simulink model "gm_CustArch_v7_vnl"  (R2020a)
settings: Solver=FixedStepDiscrete  StartTime=0.0  StopTime=840000  RelTol=1e-3
libraries: simulink x175, hdlsllib x114, hdlmdlgenlib x2
(part 2 of 4)

== system gm_CustArch_v7_vnl/cust_architecture_vnl/collect_output/read_from_magic_and_timestamp ==
  note: This subsystem in needed for save in a specific RAM the magic number
      | and the timestamp
  OutputState : Inport
  FIFO_data_in : Inport  Port=2
  FIFO_write_to : Inport  Port=3
  InputState : Inport  Port=4
  Terminator1 : Terminator
  getting address and enable for Magic and Timestamps : Subsystem
  input_RAM_for_MagicNumber_TimeStamps : hdlsllib/HDL RAMs/Dual Port RAM  ram_size=8
      settings: SourceProductBaseCode=SL
  read_from_Magic_TS : Outport
  wires:
  FIFO_write_to/1 -> getting address and enable for Magic and Timestamps/2(FIFO_write_to)
  InputState/1 -> getting address and enable for Magic and Timestamps/1(InputState)
  OutputState/1 -> input_RAM_for_MagicNumber_TimeStamps/4
  input_RAM_for_MagicNumber_TimeStamps/1 -> Terminator1/1
  getting address and enable for Magic and Timestamps/1(wr_address) -> input_RAM_for_MagicNumber_TimeStamps/2
  input_RAM_for_MagicNumber_TimeStamps/2 -> read_from_Magic_TS/1  "read_from_Magic_TS"
  getting address and enable for Magic and Timestamps/2(wr_enable) -> input_RAM_for_MagicNumber_TimeStamps/3
  FIFO_data_in/1 -> input_RAM_for_MagicNumber_TimeStamps/1

== system gm_CustArch_v7_vnl/cust_architecture_vnl/input_interpret_store_retrieve/Interpret_to_RAM_input ==
  note: These subsystems identify the sources of the incoming data (amplifier --> source_device and channel number) and
      | determine the address to be associated to the current data for the RAM storage. This statement is valid for all the kind of
      | data except for the magic number and the timestamp that are directly sent to a different RAM in the Output section
  FIFO_data_in : Inport
  FIFO_write_to : Inport  Port=2
  InputState : Inport  Port=3
  data_stream_enable : Inport  Port=4
  RAM address definition : Subsystem
  interpret incoming data : Subsystem
  device_output : Outport
  inc_source_device : Outport  Port=2
  wr_din : Outport  Port=3
  write address : Outport  Port=4
  wr_en : Outport  Port=5
  wires:
  RAM address definition/1(wr_din) -> wr_din/1  "wr_din"
  RAM address definition/2(wr_addr) -> write address/1  "write address"
  FIFO_data_in/1 -> RAM address definition/1(DataIn)
  FIFO_write_to/1 -> interpret incoming data/1(FIFO_write_to), RAM address definition/6(write_to)
  interpret incoming data/5(converter_cnt) -> RAM address definition/5(converter_cnt)
  InputState/1 -> interpret incoming data/2(InputState), RAM address definition/2(InputState)
  interpret incoming data/3(device_output) -> device_output/1
  RAM address definition/3(write_enable_6to15) -> wr_en/1  "wr_en"
  data_stream_enable/1 -> interpret incoming data/3(data_stream_enable)
  interpret incoming data/1(source_device) -> RAM address definition/4(source_device)
  interpret incoming data/2(inc_source_device) -> inc_source_device/1
  interpret incoming data/4(source_channel_0_159) -> RAM address definition/3(source_channel_0_159)

== system gm_CustArch_v7_vnl/cust_architecture_vnl/input_interpret_store_retrieve/store_and_retrieve_input ==
  note: address sent for processing
  note: data sent for processing
  note: reading address
      | from output
  note: current data
  note: current data
  note: Two dual-port RAM for storage and processing
  note: this memory is for synchronizing the current value and
      | the read_from_porcessing_addr since to ouput a value
      | the dual port RAM needs a single clock
  note: writing address
  note: data sent to Output
  read address : Inport
  wr_din : Inport  Port=2
  wr_address : Inport  Port=3
  wr_en : Inport  Port=4
  Memory4 : Memory  InheritSampleTime=on
  Terminator : Terminator
  Terminator6 : Terminator
  input_storage : hdlsllib/HDL RAMs/Dual Port RAM  ram_size=9
      settings: SourceProductBaseCode=SL
  input_storage_for_processing : hdlsllib/HDL RAMs/Dual Port RAM  ram_size=9
      settings: SourceProductBaseCode=SL
  read_from_storage_value : Outport
  current_value : Outport  Port=2
  read_from_porcessing_addr : Outport  Port=3
  wires:
  input_storage_for_processing/2 -> current_value/1  "current value"
  input_storage/2 -> read_from_storage_value/1  "read_from_storage"
  wr_din/1 -> input_storage/1, input_storage_for_processing/1
  input_storage_for_processing/1 -> Terminator6/1
  wr_en/1 -> input_storage/3, input_storage_for_processing/3
  input_storage/1 -> Terminator/1
  read address/1 -> input_storage/4
  wr_address/1 -> input_storage/2, input_storage_for_processing/2, Memory4/1
  Memory4/1 -> input_storage_for_processing/4, read_from_porcessing_addr/1  "read from porcessing addr"

== system gm_CustArch_v7_vnl/cust_architecture_vnl/output_interpret/Interpret_to_RAM_output ==
  OutputState : Inport
  data_stream_en : Inport  Port=2
  Output_State_to_RAM_address (to read) : Subsystem
  "get_enabled_timings " : Subsystem  MinMaxOverflowLogging=MinMaxAndOverflow
  rd_enable : Outport
  read address : Outport  Port=2
  wires:
  Output_State_to_RAM_address (to read)/1(rd_enable) -> rd_enable/1
  data_stream_en/1 -> "get_enabled_timings "/2(data_stream_en)
  OutputState/1 -> "get_enabled_timings "/1(OutputState), Output_State_to_RAM_address (to read)/3(OutputState)
  "get_enabled_timings "/1(source_channel_en) -> Output_State_to_RAM_address (to read)/1(source_channel_en)
  "get_enabled_timings "/2(source_channel_0_159) -> Output_State_to_RAM_address (to read)/2(source_channel_0_159)
  "get_enabled_timings "/3(source_device_enabled) -> Output_State_to_RAM_address (to read)/4(source_device_en)
  Output_State_to_RAM_address (to read)/2(rd_addr) -> read address/1
  "get_enabled_timings "/4(source_device) -> Output_State_to_RAM_address (to read)/5(source_device)
  "get_enabled_timings "/5(converter_cnt) -> Output_State_to_RAM_address (to read)/6(converter_cnt)

== system gm_CustArch_v7_vnl/cust_architecture_vnl/process_and_retrieve/digital_filter ==
  current_sample : Inport  OutDataTypeStr=fixdt(0,16,0)
  previous_sample : Inport  Port=2
  Enable : EnablePort
  Constant : Constant  Value=32768  OutDataTypeStr=fixdt(0,16,0)  SampleTime=-1
  Constant1 : Constant  Value=32768  OutDataTypeStr=fixdt(0,16,0)  SampleTime=-1
  HP_Butter_2nd : Subsystem  Tag=FilterWizardSubSystem
      settings: ErrorFcn=dspFilterRealizedInBasicElemsAlgLoopErrFcnCallback
  Subtract : Sum  Inputs=+-  OutDataTypeStr=fixdt(1,16,4)
  Subtract1 : Sum  OutDataTypeStr=fixdt(0,16,0)
  filter_output : Outport  InitialOutput=[0]
  new_previous_sample : Outport  Port=2  InitialOutput=[0]
  wires:
  HP_Butter_2nd/2(Output1) -> new_previous_sample/1
  previous_sample/1 -> HP_Butter_2nd/2(Input1)
  Subtract1/1 -> filter_output/1
  Constant1/1 -> Subtract1/2
  HP_Butter_2nd/1(Output) -> Subtract1/1
  current_sample/1 -> Subtract/1
  Subtract/1 -> HP_Butter_2nd/1(Input)
  Constant/1 -> Subtract/2

== system gm_CustArch_v7_vnl/cust_architecture_vnl/process_and_retrieve/previous_sample_storage1 ==
  note: ritardo scrittura su data2 1 campione
  new_previous_sample : Inport
  input_state_AC_TRUE-3 : Inport  Port=2
  write porcessing addr = read from storage addr +1 : Inport  Port=3
  input_state_AC_TRUE : Inport  Port=4
  1st : Constant  OutDataTypeStr=boolean  SampleTime=-1
  Bit Concat : hdlsllib/Logic and Bit Operations/Bit Concat  numInputs=2
  Compare To Constant2 : simulink/Logic and Bit Operations/Compare To Constant  relop===  const=1  OutDataTypeStr=boolean
  Delay1 : Delay  DelayLength=1  InitialCondition=0
  Delay4 : Delay  DelayLength=1  InitialCondition=0
  Mux : Mux  Inputs=2
  PreviousData1_storage : hdlsllib/HDL RAMs/Dual Port RAM  ram_size=10
      settings: SourceProductBaseCode=SL
  PreviousData1_storage1 : hdlsllib/HDL RAMs/Dual Port RAM  ram_size=10
      settings: SourceProductBaseCode=SL
  PreviousData_read : Subsystem
  ReadingStateMachine : Stateflow chart  TreatAsAtomicUnit=on
  Terminator1 : Terminator
  Terminator2 : Terminator
  previous_sample : Outport
  wires:
  Delay1/1 -> PreviousData1_storage1/2
  Delay4/1 -> PreviousData1_storage1/3
  PreviousData1_storage1/1 -> Terminator2/1
  Mux/1 -> previous_sample/1
  PreviousData1_storage1/2 -> Mux/1
  Compare To Constant2/1 -> Delay4/1, PreviousData_read/Enable
  ReadingStateMachine/1(StarReading) -> Compare To Constant2/1
  input_state_AC_TRUE/1 -> ReadingStateMachine/1(read_enable)
  PreviousData_read/1(y) -> PreviousData1_storage/4, PreviousData1_storage1/4
  write porcessing addr = read from storage addr +1/1 -> PreviousData_read/1(u2), Bit Concat/2
  input_state_AC_TRUE-3/1 -> PreviousData1_storage/3
  1st/1 -> Bit Concat/1
  PreviousData1_storage/2 -> Mux/2, PreviousData1_storage1/1
  new_previous_sample/1 -> PreviousData1_storage/1
  PreviousData1_storage/1 -> Terminator1/1
  Bit Concat/1 -> PreviousData1_storage/2, Delay1/1

== system gm_CustArch_v7_vnl/cust_architecture_vnl/process_and_retrieve/previous_sample_storage2 ==
  note: ritardo scrittura su data2 1 campione
  new_previous_sample : Inport
  input_state_AC_TRUE : Inport  Port=2
  write porcessing addr = read from storage addr +1 : Inport  Port=3
  1st : Constant  OutDataTypeStr=boolean  SampleTime=-1
  Bit Concat : hdlsllib/Logic and Bit Operations/Bit Concat  numInputs=2
  Constant : Constant  Value=0  OutDataTypeStr=boolean  SampleTime=-1
  Delay : Delay  DelayLength=3  InitialCondition=0
  Delay{1..2,4..5} (4 alike) : Delay  DelayLength=1  InitialCondition=0
  Delay3 : Delay  DelayLength=3  InitialCondition=0
  Detect Change : simulink/Logic and Bit Operations/Detect Change  vinit=0  OutDataTypeStr=boolean
  Mux : Mux  Inputs=2
  PreviousData1_storage : hdlsllib/HDL RAMs/Dual Port RAM  ram_size=10
      settings: SourceProductBaseCode=SL
  PreviousData1_storage1 : hdlsllib/HDL RAMs/Dual Port RAM  ram_size=10
      settings: SourceProductBaseCode=SL
  PreviousData_read : Subsystem
  ReadingStateMachine : Stateflow chart  Commented=on  TreatAsAtomicUnit=on
  Switch : Switch  Criteria=u2 > Threshold
  Terminator1 : Terminator
  Terminator2 : Terminator
  previous_sample : Outport
  wires:
  Switch/1 -> PreviousData1_storage/4, PreviousData1_storage1/4, Delay4/1
  PreviousData_read/1(y) -> Detect Change/1, Switch/1
  Detect Change/1 -> Switch/2
  Constant/1 -> Switch/3
  Mux/1 -> previous_sample/1
  PreviousData1_storage1/2 -> Mux/1
  Delay5/1 -> PreviousData1_storage1/3
  PreviousData1_storage/2 -> PreviousData1_storage1/1, Mux/2
  PreviousData1_storage1/1 -> Terminator2/1
  Delay4/1 -> PreviousData1_storage1/2
  Delay3/1 -> Bit Concat/2
  Delay2/1 -> PreviousData_read/1(u2)
  Delay1/1 -> PreviousData_read/Enable, Delay5/1
  Delay/1 -> PreviousData1_storage/3
  write porcessing addr = read from storage addr +1/1 -> Delay3/1, Delay2/1
  input_state_AC_TRUE/1 -> Delay/1, Delay1/1
  1st/1 -> Bit Concat/1
  new_previous_sample/1 -> PreviousData1_storage/1
  PreviousData1_storage/1 -> Terminator1/1
  Bit Concat/1 -> PreviousData1_storage/2

== system gm_CustArch_v7_vnl/cust_architecture/collect_output/read_from_magic_and_timestamp/getting address and enable for Magic and Timestamps ==
  note: enable the RAM writing if the InputState is between 0 and 5
  InputState : Inport  OutDataTypeStr=uint8  PortDimensions=1  SampleTime=1
  FIFO_write_to : Inport  Port=2  OutDataTypeStr=boolean  PortDimensions=1  SampleTime=1
  AND1 : Logic  AllPortsSameDT=off  OutDataTypeStr=boolean  SampleTime=1
  Compare To Constant10 : simulink/Logic and Bit Operations/Compare To Constant  relop===  const="fi(0,0,8,0,\"hex\",\"04\")"  OutDataTypeStr=boolean
  Compare To Constant11 : simulink/Logic and Bit Operations/Compare To Constant  relop===  const="fi(0,0,8,0,\"hex\",\"05\")"  OutDataTypeStr=boolean
  Compare To Constant12 : simulink/Logic and Bit Operations/Compare To Constant  relop=<=  const="fi(0,0,8,0,\"hex\",\"05\")"  OutDataTypeStr=boolean
  Compare To Constant6 : simulink/Logic and Bit Operations/Compare To Constant  relop===  const="fi(0,0,8,0,\"hex\",\"00\")"  OutDataTypeStr=boolean
  Compare To Constant7 : simulink/Logic and Bit Operations/Compare To Constant  relop===  const="fi(0,0,8,0,\"hex\",\"01\")"  OutDataTypeStr=boolean
  Compare To Constant8 : simulink/Logic and Bit Operations/Compare To Constant  relop===  const="fi(0,0,8,0,\"hex\",\"02\")"  OutDataTypeStr=boolean
  Compare To Constant9 : simulink/Logic and Bit Operations/Compare To Constant  relop===  const="fi(0,0,8,0,\"hex\",\"03\")"  OutDataTypeStr=boolean
  Constant10 : Constant  Value=3  OutDataTypeStr=uint8  SampleTime=1
  Constant11 : Constant  Value=4  OutDataTypeStr=uint8  SampleTime=1
  Constant12 : Constant  Value=5  OutDataTypeStr=uint8  SampleTime=1
  Constant13 : Constant  Value=6  OutDataTypeStr=uint8  SampleTime=1
  Constant7 : Constant  Value=0  OutDataTypeStr=uint8  SampleTime=1
  Constant8 : Constant  OutDataTypeStr=uint8  SampleTime=1
  Constant9 : Constant  Value=2  OutDataTypeStr=uint8  SampleTime=1
  Switch{6..11} (6 alike) : Switch  Criteria=u2 > Threshold  Threshold=double(0)  OutDataTypeStr=uint8  SampleTime=1
  wr_address : Outport  VectorParamsAs1DForOutWhenUnconnected=off
  wr_enable : Outport  Port=2  VectorParamsAs1DForOutWhenUnconnected=off
  wires:
  Switch9/1 -> Switch8/3
  Switch8/1 -> Switch7/3
  Switch7/1 -> Switch6/3
  Switch6/1 -> wr_address/1
  Switch11/1 -> Switch10/3
  Switch10/1 -> Switch9/3
  Constant9/1 -> Switch8/1
  Constant8/1 -> Switch7/1
  Constant7/1 -> Switch6/1
  Constant13/1 -> Switch11/3
  Constant12/1 -> Switch11/1
  Constant11/1 -> Switch10/1
  Constant10/1 -> Switch9/1
  Compare To Constant9/1 -> Switch9/2
  Compare To Constant8/1 -> Switch8/2
  Compare To Constant7/1 -> Switch7/2
  Compare To Constant6/1 -> Switch6/2
  Compare To Constant12/1 -> AND1/1
  Compare To Constant11/1 -> Switch11/2
  Compare To Constant10/1 -> Switch10/2
  AND1/1 -> wr_enable/1
  FIFO_write_to/1 -> AND1/2
  InputState/1 -> Compare To Constant10/1, Compare To Constant11/1, Compare To Constant12/1, Compare To Constant6/1, Compare To Constant7/1, Compare To Constant8/1, Compare To Constant9/1

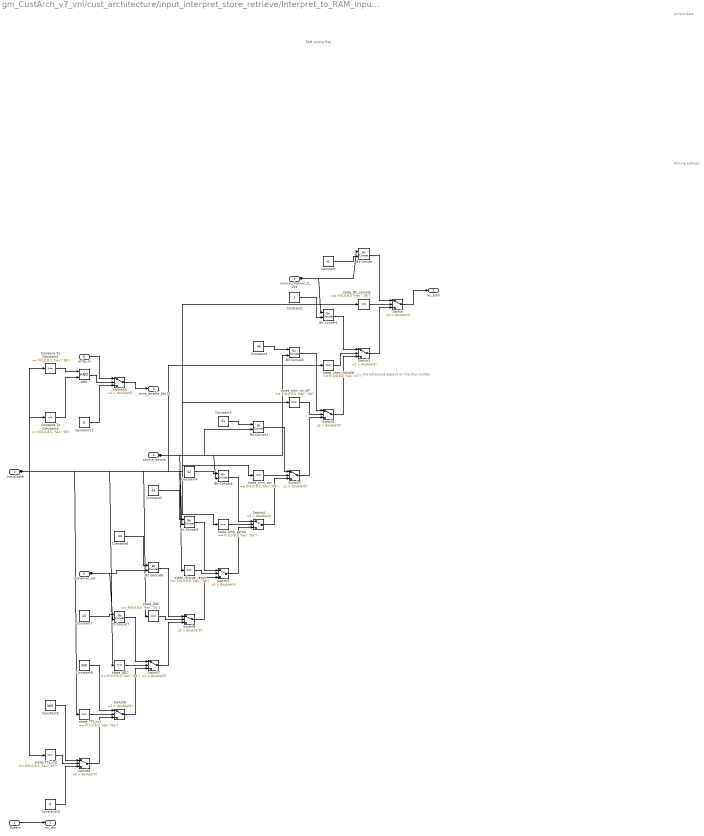
== system gm_CustArch_v7_vnl/cust_architecture/input_interpret_store_retrieve/Interpret_to_RAM_input/RAM address definition ==
  note: RAM writing flag
  note: current data
  note: Writing address
  note: the adressess depend on the chip number
  DataIn : Inport  OutDataTypeStr=uint16  PortDimensions=1  SampleTime=1
  InputState : Inport  Port=2  OutDataTypeStr=uint8  PortDimensions=1  SampleTime=1
  source_channel_0_159 : Inport  Port=3  OutDataTypeStr=uint8  PortDimensions=1  SampleTime=1
  source_device : Inport  Port=4  OutDataTypeStr=fixdt(0, 3, 0)  PortDimensions=1  SampleTime=1
  converter_cnt : Inport  Port=5  OutDataTypeStr=fixdt(0, 3, 0)  PortDimensions=1  SampleTime=1
  write_to : Inport  Port=6  OutDataTypeStr=boolean  PortDimensions=1  SampleTime=1
  AND : Logic  AllPortsSameDT=off  OutDataTypeStr=boolean  SampleTime=1
  Bit Concat{,1..7} (8 alike) : hdlsllib/Logic and Bit Operations/Bit Concat  numInputs=2
  Compare To Constant2 : simulink/Logic and Bit Operations/Compare To Constant  relop=>=  const="fi(0,0,8,0,\"hex\",\"06\")"  OutDataTypeStr=boolean
  Compare To Constant3 : simulink/Logic and Bit Operations/Compare To Constant  relop=<=  const="fi(0,0,8,0,\"hex\",\"0f\")"  OutDataTypeStr=boolean
  Constant : Constant  Value=0  OutDataTypeStr=boolean  SampleTime=1
  Constant1 : Constant  OutDataTypeStr=boolean  SampleTime=1
  Constant10 : Constant  Value=0  OutDataTypeStr=fixdt(0, 9, 1000)  SampleTime=1
  Constant11 : Constant  Value=0  OutDataTypeStr=boolean  SampleTime=1
  Constant2 : Constant  Value=40  OutDataTypeStr=fixdt(0, 6, 0)  SampleTime=1
  Constant3 : Constant  Value=41  OutDataTypeStr=fixdt(0, 6, 0)  SampleTime=1
  Constant4 : Constant  Value=42  OutDataTypeStr=fixdt(0, 6, 0)  SampleTime=1
  Constant5 : Constant  Value=43  OutDataTypeStr=fixdt(0, 6, 0)  SampleTime=1
  Constant6 : Constant  Value=44  OutDataTypeStr=fixdt(0, 6, 0)  SampleTime=1
  Constant7 : Constant  Value=45  OutDataTypeStr=fixdt(0, 6, 0)  SampleTime=1
  Constant8 : Constant  Value=368  OutDataTypeStr=fixdt(0, 9, 0)  SampleTime=1
  Constant9 : Constant  Value=369  OutDataTypeStr=fixdt(0, 9, 0)  SampleTime=1
  Switch{,1..9} (10 alike) : Switch  Criteria=u2 > Threshold  Threshold=double(0)  OutDataTypeStr=fixdt(0, 9, 0)  SampleTime=1
  Switch10 : Switch  Criteria=u2 > Threshold  Threshold=double(0)  OutDataTypeStr=boolean  SampleTime=1
  state_ADC : simulink/Logic and Bit Operations/Compare To Constant  relop===  const="fi(0,0,8,0,\"hex\",\"0d\")"  OutDataTypeStr=boolean
  state_DAC : simulink/Logic and Bit Operations/Compare To Constant  relop===  const="fi(0,0,8,0,\"hex\",\"0c\")"  OutDataTypeStr=boolean
  state_DC_sample : simulink/Logic and Bit Operations/Compare To Constant  relop===  const="fi(0,0,8,0,\"hex\",\"06\")"  OutDataTypeStr=boolean
  state_TTL_in1 : simulink/Logic and Bit Operations/Compare To Constant  relop===  const="fi(0,0,8,0,\"hex\",\"0e\")"  OutDataTypeStr=boolean
  state_TTL_in2 : simulink/Logic and Bit Operations/Compare To Constant  relop===  const="fi(0,0,8,0,\"hex\",\"0f\")"  OutDataTypeStr=boolean
  state_amp_settle : simulink/Logic and Bit Operations/Compare To Constant  relop===  const="fi(0,0,8,0,\"hex\",\"0a\")"  OutDataTypeStr=boolean
  state_chan_sample : simulink/Logic and Bit Operations/Compare To Constant  relop===  const="fi(0,0,8,0,\"hex\",\"07\")"  OutDataTypeStr=boolean
  state_charge_recov : simulink/Logic and Bit Operations/Compare To Constant  relop===  const="fi(0,0,8,0,\"hex\",\"0b\")"  OutDataTypeStr=boolean
  state_stim_on_off : simulink/Logic and Bit Operations/Compare To Constant  relop===  const="fi(0,0,8,0,\"hex\",\"08\")"  OutDataTypeStr=boolean
  state_stim_pol : simulink/Logic and Bit Operations/Compare To Constant  relop===  const="fi(0,0,8,0,\"hex\",\"09\")"  OutDataTypeStr=boolean
  wr_din : Outport  VectorParamsAs1DForOutWhenUnconnected=off
  wr_addr : Outport  Port=2  OutDataTypeStr=fixdt(0,9,0)  VectorParamsAs1DForOutWhenUnconnected=off
  write_enable_6to15 : Outport  Port=3  OutDataTypeStr=boolean  VectorParamsAs1DForOutWhenUnconnected=off
  wires:
  state_stim_pol/1 -> Switch3/2
  state_stim_on_off/1 -> Switch2/2
  state_charge_recov/1 -> Switch5/2
  state_chan_sample/1 -> Switch1/2
  state_amp_settle/1 -> Switch4/2
  state_TTL_in2/1 -> Switch9/2
  state_TTL_in1/1 -> Switch8/2
  state_DC_sample/1 -> Switch/2
  state_DAC/1 -> Switch6/2
  state_ADC/1 -> Switch7/2
  Switch9/1 -> Switch8/3
  Switch8/1 -> Switch7/3
  Switch7/1 -> Switch6/3
  Switch6/1 -> Switch5/3
  Switch5/1 -> Switch4/3
  Switch4/1 -> Switch3/3
  Switch3/1 -> Switch2/3
  Switch2/1 -> Switch1/3
  Switch10/1 -> write_enable_6to15/1
  Switch1/1 -> Switch/3
  Switch/1 -> wr_addr/1
  Constant9/1 -> Switch9/1
  Constant8/1 -> Switch8/1
  Constant7/1 -> Bit Concat7/1
  Constant6/1 -> Bit Concat6/1
  Constant5/1 -> Bit Concat5/1
  Constant4/1 -> Bit Concat4/1
  Constant3/1 -> Bit Concat3/1
  Constant2/1 -> Bit Concat2/1
  Constant11/1 -> Switch10/3
  Constant10/1 -> Switch9/3
  Constant1/1 -> Bit Concat1/2
  Constant/1 -> Bit Concat/2
  Compare To Constant3/1 -> AND/2
  Compare To Constant2/1 -> AND/1
  Bit Concat7/1 -> Switch7/1
  Bit Concat6/1 -> Switch6/1
  Bit Concat5/1 -> Switch5/1
  Bit Concat4/1 -> Switch4/1
  Bit Concat3/1 -> Switch3/1
  Bit Concat2/1 -> Switch2/1
  Bit Concat1/1 -> Switch1/1
  Bit Concat/1 -> Switch/1
  AND/1 -> Switch10/2
  write_to/1 -> Switch10/1
  converter_cnt/1 -> Bit Concat6/2, Bit Concat7/2
  source_device/1 -> Bit Concat2/2, Bit Concat3/2, Bit Concat4/2, Bit Concat5/2
  source_channel_0_159/1 -> Bit Concat/1, Bit Concat1/1
  InputState/1 -> Compare To Constant2/1, Compare To Constant3/1, state_ADC/1, state_DAC/1, state_DC_sample/1, state_TTL_in1/1, state_TTL_in2/1, state_amp_settle/1, state_chan_sample/1, state_charge_recov/1, state_stim_on_off/1, state_stim_pol/1
  DataIn/1 -> wr_din/1

== system gm_CustArch_v7_vnl/cust_architecture/input_interpret_store_retrieve/Interpret_to_RAM_input/interpret incoming data ==
  note: counter of the converters
  note: check ADC/DAC state
  FIFO_write_to : Inport  OutDataTypeStr=boolean  PortDimensions=1  SampleTime=1
  InputState : Inport  Port=2  OutDataTypeStr=uint8  PortDimensions=1  SampleTime=1
  data_stream_enable : Inport  Port=3  OutDataTypeStr=uint8  PortDimensions=1  SampleTime=1
  Bit Slice : hdlsllib/Logic and Bit Operations/Bit Slice  lidx=double(2)  ridx=double(0)
      settings: SourceProductBaseCode=SL
  Bit Slice1 : hdlsllib/Logic and Bit Operations/Bit Slice  lidx=double(2)  ridx=double(0)
      settings: SourceProductBaseCode=SL
  HDL Counter : hdlsllib/Sources/HDL Counter  CountType=Count limited  CountInit=double(0)  CountStep=double(1)  CountMax=double(7)  CountFromType=Initial value  CountFrom=double(0)  CountResetPort=off  CountLoadPort=off  CountEnbPort=on  CountDirPort=off  CountDataType=Unsigned  CountWordLen=8  CountFracLen=0  CountSampTime=1
  "condition to count DAC or ADC " : Subsystem
  get_sources_and_RAM_addresses : Subsystem
  source_device : Outport  VectorParamsAs1DForOutWhenUnconnected=off
  inc_source_device : Outport  Port=2  VectorParamsAs1DForOutWhenUnconnected=off
  device_output : Outport  Port=3  VectorParamsAs1DForOutWhenUnconnected=off
  source_channel_0_159 : Outport  Port=4  VectorParamsAs1DForOutWhenUnconnected=off
  converter_cnt : Outport  Port=5  VectorParamsAs1DForOutWhenUnconnected=off
  wires:
  get_sources_and_RAM_addresses/4(inc_source_device) -> inc_source_device/1
  get_sources_and_RAM_addresses/3(source_channel) -> source_channel_0_159/1
  get_sources_and_RAM_addresses/2(device_output) -> device_output/1
  get_sources_and_RAM_addresses/1(source_device) -> Bit Slice1/1
  "condition to count DAC or ADC "/1(Out1) -> HDL Counter/1
  HDL Counter/1 -> Bit Slice/1
  Bit Slice1/1 -> source_device/1
  Bit Slice/1 -> converter_cnt/1
  data_stream_enable/1 -> get_sources_and_RAM_addresses/3(data_stream_enable)
  InputState/1 -> get_sources_and_RAM_addresses/2(InputState), "condition to count DAC or ADC "/2(input_state)
  FIFO_write_to/1 -> get_sources_and_RAM_addresses/1(FIFO_write_to), "condition to count DAC or ADC "/1(fifo_write_to)

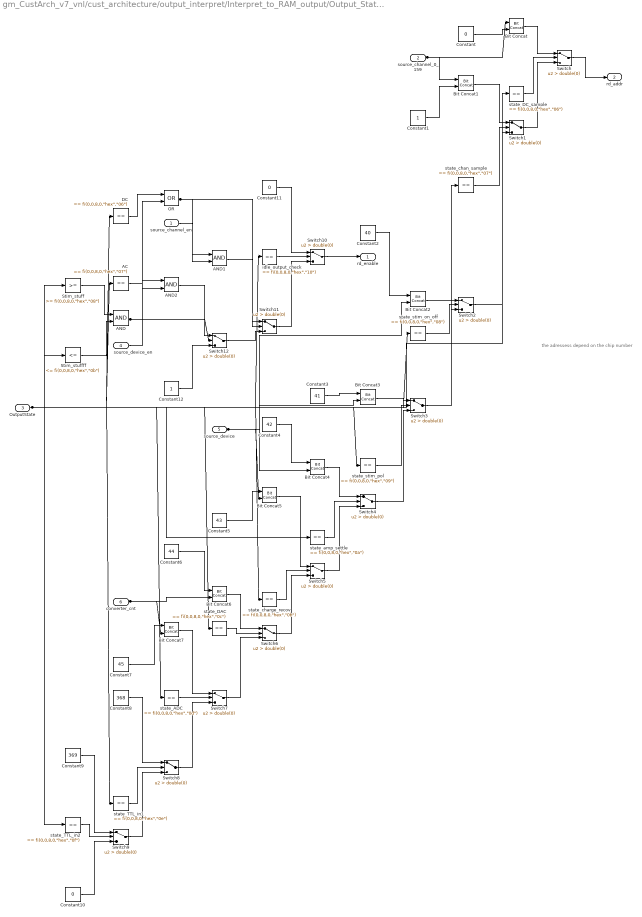
== system gm_CustArch_v7_vnl/cust_architecture/output_interpret/Interpret_to_RAM_output/Output_State_to_RAM_address (to read) ==
  note: the adressess depend on the chip number
  source_channel_en : Inport  OutDataTypeStr=boolean  PortDimensions=1  SampleTime=1
  source_channel_0_159 : Inport  Port=2  OutDataTypeStr=uint8  PortDimensions=1  SampleTime=1
  OutputState : Inport  Port=3  OutDataTypeStr=uint8  PortDimensions=1  SampleTime=1
  source_device_en : Inport  Port=4  OutDataTypeStr=fixdt(0, 1, 0)  PortDimensions=1  SampleTime=1
  source_device : Inport  Port=5  OutDataTypeStr=fixdt(0, 3, 0)  PortDimensions=1  SampleTime=1
  converter_cnt : Inport  Port=6  OutDataTypeStr=fixdt(0, 3, 0)  PortDimensions=1  SampleTime=1
  AC : simulink/Logic and Bit Operations/Compare To Constant  relop===  const="fi(0,0,8,0,\"hex\",\"07\")"  OutDataTypeStr=boolean
  AND : Logic  AllPortsSameDT=off  OutDataTypeStr=boolean  SampleTime=1
  AND1 : Logic  AllPortsSameDT=off  OutDataTypeStr=boolean  SampleTime=1
  AND2 : Logic  AllPortsSameDT=off  OutDataTypeStr=boolean  SampleTime=1
  Bit Concat{,1..7} (8 alike) : hdlsllib/Logic and Bit Operations/Bit Concat  numInputs=2
  Constant : Constant  Value=0  OutDataTypeStr=boolean  SampleTime=1
  Constant1 : Constant  OutDataTypeStr=boolean  SampleTime=1
  Constant10 : Constant  Value=0  OutDataTypeStr=fixdt(0, 9, 1000)  SampleTime=1
  Constant11 : Constant  Value=0  OutDataTypeStr=boolean  SampleTime=1
  Constant12 : Constant  OutDataTypeStr=boolean  SampleTime=1
  Constant2 : Constant  Value=40  OutDataTypeStr=fixdt(0, 6, 0)  SampleTime=1
  Constant3 : Constant  Value=41  OutDataTypeStr=fixdt(0, 6, 0)  SampleTime=1
  Constant4 : Constant  Value=42  OutDataTypeStr=fixdt(0, 6, 0)  SampleTime=1
  Constant5 : Constant  Value=43  OutDataTypeStr=fixdt(0, 6, 0)  SampleTime=1
  Constant6 : Constant  Value=44  OutDataTypeStr=fixdt(0, 6, 0)  SampleTime=1
  Constant7 : Constant  Value=45  OutDataTypeStr=fixdt(0, 6, 0)  SampleTime=1
  Constant8 : Constant  Value=368  OutDataTypeStr=fixdt(0, 9, 0)  SampleTime=1
  Constant9 : Constant  Value=369  OutDataTypeStr=fixdt(0, 9, 0)  SampleTime=1
  DC : simulink/Logic and Bit Operations/Compare To Constant  relop===  const="fi(0,0,8,0,\"hex\",\"06\")"  OutDataTypeStr=boolean
  OR : Logic  Operator=OR  AllPortsSameDT=off  OutDataTypeStr=boolean  SampleTime=1
  Stim_stuff : simulink/Logic and Bit Operations/Compare To Constant  relop=>=  const="fi(0,0,8,0,\"hex\",\"08\")"  OutDataTypeStr=boolean
  Stim_stuffff : simulink/Logic and Bit Operations/Compare To Constant  relop=<=  const="fi(0,0,8,0,\"hex\",\"0b\")"  OutDataTypeStr=boolean
  Switch{,1..9} (10 alike) : Switch  Criteria=u2 > Threshold  Threshold=double(0)  OutDataTypeStr=fixdt(0, 9, 0)  SampleTime=1
  Switch10 : Switch  Criteria=u2 > Threshold  Threshold=double(0)  OutDataTypeStr=boolean  SampleTime=1
  Switch11 : Switch  Criteria=u2 > Threshold  Threshold=double(0)  OutDataTypeStr=boolean  SampleTime=1
  Switch12 : Switch  Criteria=u2 > Threshold  Threshold=double(0)  OutDataTypeStr=boolean  SampleTime=1
  idle_output_check : simulink/Logic and Bit Operations/Compare To Constant  relop===  const="fi(0,0,8,0,\"hex\",\"10\")"  OutDataTypeStr=boolean
  state_ADC : simulink/Logic and Bit Operations/Compare To Constant  relop===  const="fi(0,0,8,0,\"hex\",\"0d\")"  OutDataTypeStr=boolean
  state_DAC : simulink/Logic and Bit Operations/Compare To Constant  relop===  const="fi(0,0,8,0,\"hex\",\"0c\")"  OutDataTypeStr=boolean
  state_DC_sample : simulink/Logic and Bit Operations/Compare To Constant  relop===  const="fi(0,0,8,0,\"hex\",\"06\")"  OutDataTypeStr=boolean
  state_TTL_in1 : simulink/Logic and Bit Operations/Compare To Constant  relop===  const="fi(0,0,8,0,\"hex\",\"0e\")"  OutDataTypeStr=boolean
  state_TTL_in2 : simulink/Logic and Bit Operations/Compare To Constant  relop===  const="fi(0,0,8,0,\"hex\",\"0f\")"  OutDataTypeStr=boolean
  state_amp_settle : simulink/Logic and Bit Operations/Compare To Constant  relop===  const="fi(0,0,8,0,\"hex\",\"0a\")"  OutDataTypeStr=boolean
  state_chan_sample : simulink/Logic and Bit Operations/Compare To Constant  relop===  const="fi(0,0,8,0,\"hex\",\"07\")"  OutDataTypeStr=boolean
  state_charge_recov : simulink/Logic and Bit Operations/Compare To Constant  relop===  const="fi(0,0,8,0,\"hex\",\"0b\")"  OutDataTypeStr=boolean
  state_stim_on_off : simulink/Logic and Bit Operations/Compare To Constant  relop===  const="fi(0,0,8,0,\"hex\",\"08\")"  OutDataTypeStr=boolean
  state_stim_pol : simulink/Logic and Bit Operations/Compare To Constant  relop===  const="fi(0,0,8,0,\"hex\",\"09\")"  OutDataTypeStr=boolean
  rd_enable : Outport  VectorParamsAs1DForOutWhenUnconnected=off
  rd_addr : Outport  Port=2  OutDataTypeStr=fixdt(0,9,0)  VectorParamsAs1DForOutWhenUnconnected=off
  wires:
  state_stim_pol/1 -> Switch3/2
  state_stim_on_off/1 -> Switch2/2
  state_charge_recov/1 -> Switch5/2
  state_chan_sample/1 -> Switch1/2
  state_amp_settle/1 -> Switch4/2
  state_TTL_in2/1 -> Switch9/2
  state_TTL_in1/1 -> Switch8/2
  state_DC_sample/1 -> Switch/2
  state_DAC/1 -> Switch6/2
  state_ADC/1 -> Switch7/2
  idle_output_check/1 -> Switch10/2
  Switch9/1 -> Switch8/3
  Switch8/1 -> Switch7/3
  Switch7/1 -> Switch6/3
  Switch6/1 -> Switch5/3
  Switch5/1 -> Switch4/3
  Switch4/1 -> Switch3/3
  Switch3/1 -> Switch2/3
  Switch2/1 -> Switch1/3
  Switch12/1 -> Switch11/3
  Switch11/1 -> Switch10/3
  Switch10/1 -> rd_enable/1
  Switch1/1 -> Switch/3
  Switch/1 -> rd_addr/1
  Stim_stuffff/1 -> AND/2
  Stim_stuff/1 -> AND/1
  OR/1 -> AND1/1, Switch11/2
  DC/1 -> OR/1
  Constant9/1 -> Switch9/1
  Constant8/1 -> Switch8/1
  Constant7/1 -> Bit Concat7/1
  Constant6/1 -> Bit Concat6/1
  Constant5/1 -> Bit Concat5/1
  Constant4/1 -> Bit Concat4/1
  Constant3/1 -> Bit Concat3/1
  Constant2/1 -> Bit Concat2/1
  Constant12/1 -> Switch12/3
  Constant11/1 -> Switch10/1
  Constant10/1 -> Switch9/3
  Constant1/1 -> Bit Concat1/2
  Constant/1 -> Bit Concat/2
  Bit Concat7/1 -> Switch7/1
  Bit Concat6/1 -> Switch6/1
  Bit Concat5/1 -> Switch5/1
  Bit Concat4/1 -> Switch4/1
  Bit Concat3/1 -> Switch3/1
  Bit Concat2/1 -> Switch2/1
  Bit Concat1/1 -> Switch1/1
  Bit Concat/1 -> Switch/1
  AND2/1 -> Switch12/1
  AND1/1 -> Switch11/1
  AND/1 -> AND2/1, Switch12/2
  AC/1 -> OR/2
  converter_cnt/1 -> Bit Concat6/2, Bit Concat7/2
  source_device/1 -> Bit Concat2/2, Bit Concat3/2, Bit Concat4/2, Bit Concat5/2
  source_device_en/1 -> AND2/2
  OutputState/1 -> AC/1, DC/1, Stim_stuff/1, Stim_stuffff/1, idle_output_check/1, state_ADC/1, state_DAC/1, state_DC_sample/1, state_TTL_in1/1, state_TTL_in2/1, state_amp_settle/1, state_chan_sample/1, state_charge_recov/1, state_stim_on_off/1, state_stim_pol/1
  source_channel_0_159/1 -> Bit Concat/1, Bit Concat1/1
  source_channel_en/1 -> AND1/2

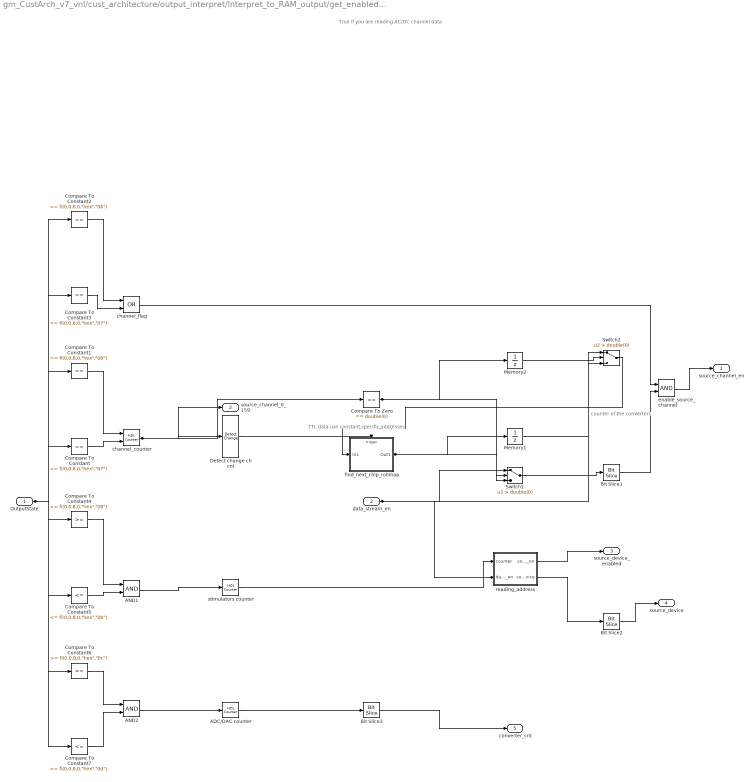
== system gm_CustArch_v7_vnl/cust_architecture/output_interpret/Interpret_to_RAM_output/get_enabled_timings  ==
  note: True if you are reading AC/DC channel data
  note: TTL data use constant specific addresses
  note: counter of the converters
  OutputState : Inport  OutDataTypeStr=uint8  PortDimensions=1  SampleTime=1
  data_stream_en : Inport  Port=2  OutDataTypeStr=uint8  PortDimensions=1  SampleTime=1
  ADC/DAC counter : hdlsllib/Sources/HDL Counter  CountType=Count limited  CountInit=double(0)  CountStep=double(1)  CountMax=double(7)  CountFromType=Initial value  CountFrom=double(0)  CountResetPort=off  CountLoadPort=off  CountEnbPort=on  CountDirPort=off  CountDataType=Unsigned  CountWordLen=8  CountFracLen=0  CountSampTime=1
  AND1 : Logic  AllPortsSameDT=off  OutDataTypeStr=boolean  SampleTime=1
  AND2 : Logic  AllPortsSameDT=off  OutDataTypeStr=boolean  SampleTime=1
  Bit Slice1 : hdlsllib/Logic and Bit Operations/Bit Slice  lidx=double(0)  ridx=double(0)
      settings: SourceProductBaseCode=SL
  Bit Slice2 : hdlsllib/Logic and Bit Operations/Bit Slice  lidx=double(2)  ridx=double(0)
      settings: SourceProductBaseCode=SL
  Bit Slice3 : hdlsllib/Logic and Bit Operations/Bit Slice  lidx=double(2)  ridx=double(0)
      settings: SourceProductBaseCode=SL
  Compare To Constant : simulink/Logic and Bit Operations/Compare To Constant  relop===  const="fi(0,0,8,0,\"hex\",\"07\")"  OutDataTypeStr=boolean
  Compare To Constant1 : simulink/Logic and Bit Operations/Compare To Constant  relop===  const="fi(0,0,8,0,\"hex\",\"08\")"  OutDataTypeStr=boolean
  Compare To Constant2 : simulink/Logic and Bit Operations/Compare To Constant  relop===  const="fi(0,0,8,0,\"hex\",\"06\")"  OutDataTypeStr=boolean
  Compare To Constant3 : simulink/Logic and Bit Operations/Compare To Constant  relop===  const="fi(0,0,8,0,\"hex\",\"07\")"  OutDataTypeStr=boolean
  Compare To Constant4 : simulink/Logic and Bit Operations/Compare To Constant  relop=>=  const="fi(0,0,8,0,\"hex\",\"08\")"  OutDataTypeStr=boolean
  Compare To Constant5 : simulink/Logic and Bit Operations/Compare To Constant  relop=<=  const="fi(0,0,8,0,\"hex\",\"0b\")"  OutDataTypeStr=boolean
  Compare To Constant6 : simulink/Logic and Bit Operations/Compare To Constant  relop=>=  const="fi(0,0,8,0,\"hex\",\"0c\")"  OutDataTypeStr=boolean
  Compare To Constant7 : simulink/Logic and Bit Operations/Compare To Constant  relop=<=  const="fi(0,0,8,0,\"hex\",\"0d\")"  OutDataTypeStr=boolean
  Compare To Zero : simulink/Logic and Bit Operations/Compare To Constant  relop===  const=double(0)  OutDataTypeStr=boolean
  Detect change ch cnt : simulink/Logic and Bit Operations/Detect Change  vinit=0  OutDataTypeStr=boolean
  Memory1 : UnitDelay  InitialCondition=double(0)  SampleTime=1
  Memory2 : UnitDelay  InitialCondition=double(0)  SampleTime=1
  Switch1 : Switch  Criteria=u2 > Threshold  Threshold=double(0)  OutDataTypeStr=uint8  SampleTime=1
  Switch2 : Switch  Criteria=u2 > Threshold  Threshold=double(0)  OutDataTypeStr=uint8  SampleTime=1
  channel_counter : hdlsllib/Sources/HDL Counter  CountType=Count limited  CountInit=double(0)  CountStep=double(1)  CountMax=double(159)  CountFromType=Initial value  CountFrom=double(0)  CountResetPort=on  CountLoadPort=off  CountEnbPort=on  CountDirPort=off  CountDataType=Unsigned  CountWordLen=8  CountFracLen=0  CountSampTime=1
  channel_flag : Logic  Operator=OR  AllPortsSameDT=off  OutDataTypeStr=boolean  SampleTime=1
  enable_source_channel : Logic  AllPortsSameDT=off  OutDataTypeStr=boolean  SampleTime=1
  find_next_chip_rollmap : Subsystem
  reading_address : Subsystem
  stimulators counter : hdlsllib/Sources/HDL Counter  CountType=Count limited  CountInit=double(0)  CountStep=double(1)  CountMax=double(7)  CountFromType=Initial value  CountFrom=double(0)  CountResetPort=off  CountLoadPort=off  CountEnbPort=on  CountDirPort=off  CountDataType=Unsigned  CountWordLen=8  CountFracLen=0  CountSampTime=1
  source_channel_en : Outport  VectorParamsAs1DForOutWhenUnconnected=off
  source_channel_0_159 : Outport  Port=2  OutMin=0  OutMax=159  OutDataTypeStr=uint8  VectorParamsAs1DForOutWhenUnconnected=off  LockScale=on
  source_device_enabled : Outport  Port=3  VectorParamsAs1DForOutWhenUnconnected=off
  source_device : Outport  Port=4  VectorParamsAs1DForOutWhenUnconnected=off
  converter_cnt : Outport  Port=5  VectorParamsAs1DForOutWhenUnconnected=off
  wires:
  stimulators counter/1 -> reading_address/1("counter ")
  reading_address/2(source_device) -> Bit Slice2/1
  reading_address/1(source_device_en) -> source_device_enabled/1
  find_next_chip_rollmap/1(Out1) -> Memory1/1, Switch1/3
  enable_source_channel/1 -> source_channel_en/1
  channel_flag/1 -> enable_source_channel/1
  channel_counter/1 -> source_channel_0_159/1, Detect change ch cnt/1, Compare To Zero/1
  Switch2/1 -> find_next_chip_rollmap/1(In1)
  Switch1/1 -> Bit Slice1/1
  Memory2/1 -> Switch2/2
  Memory1/1 -> Switch2/3
  Detect change ch cnt/1 -> find_next_chip_rollmap/Trigger
  Compare To Zero/1 -> Memory2/1, Switch1/2
  Compare To Constant7/1 -> AND2/2
  Compare To Constant6/1 -> AND2/1
  Compare To Constant5/1 -> AND1/2
  Compare To Constant4/1 -> AND1/1
  Compare To Constant3/1 -> channel_flag/2
  Compare To Constant2/1 -> channel_flag/1
  Compare To Constant1/1 -> channel_counter/1
  Compare To Constant/1 -> channel_counter/2
  Bit Slice3/1 -> converter_cnt/1
  Bit Slice2/1 -> source_device/1
  Bit Slice1/1 -> enable_source_channel/2
  AND2/1 -> ADC/DAC counter/1
  AND1/1 -> stimulators counter/1
  ADC/DAC counter/1 -> Bit Slice3/1
  data_stream_en/1 -> reading_address/2(data_stream_en), Switch1/1, Switch2/1
  OutputState/1 -> Compare To Constant/1, Compare To Constant1/1, Compare To Constant2/1, Compare To Constant3/1, Compare To Constant4/1, Compare To Constant5/1, Compare To Constant6/1, Compare To Constant7/1

== system gm_CustArch_v7_vnl/cust_architecture/process_and_retrieve/digital_filter/HP_Butter_2nd ==
  Input : Inport  OutDataTypeStr=fixdt(1, 16, 4)  PortDimensions=1  SampleTime=1
  Input1 : Inport  Port=2  OutDataTypeStr=fixdt(1, 16, -2)  PortDimensions=[2]  SampleTime=1
  CastState1 : DataTypeConversion  OutDataTypeStr=fixdt(1, 16, -2)  RndMeth=Convergent  SampleTime=1  SaturateOnIntegerOverflow=on
  ConvertIn : DataTypeConversion  OutDataTypeStr=fixdt(1, 16, 4)  RndMeth=Nearest  SampleTime=1  SaturateOnIntegerOverflow=on
  ConvertOut : DataTypeConversion  OutDataTypeStr=fixdt(1, 16, 5)  RndMeth=Convergent  SampleTime=1  SaturateOnIntegerOverflow=on
  Input1_0_wire : hdlmdlgenlib/Buffer
      settings: SourceProductBaseCode=SL
  Input1_1_wire : hdlmdlgenlib/Buffer
      settings: SourceProductBaseCode=SL
  SumA21 : Sum  Inputs=+-  AccumDataTypeStr=fixdt(1, 34, 15)  OutDataTypeStr=fixdt(1, 34, 15)  RndMeth=Convergent  SaturateOnIntegerOverflow=on  SampleTime=1
  SumA31 : Sum  Inputs=+-  AccumDataTypeStr=fixdt(1, 34, 15)  OutDataTypeStr=fixdt(1, 34, 16)  RndMeth=Convergent  SaturateOnIntegerOverflow=on  SampleTime=1
  SumB21 : Sum  AccumDataTypeStr=fixdt(1, 34, 15)  OutDataTypeStr=fixdt(1, 34, 16)  RndMeth=Convergent  SaturateOnIntegerOverflow=on  SampleTime=1
  SumB31 : Sum  AccumDataTypeStr=fixdt(1, 34, 16)  OutDataTypeStr=fixdt(1, 34, 23)  RndMeth=Convergent  SaturateOnIntegerOverflow=on  SampleTime=1
  a(2)(1) : Gain  Gain="fi(0,1,16,14,\"hex\",\"85af\")"  ParamDataTypeStr=fixdt(1, 16, 14)  OutDataTypeStr=fixdt(1, 32, 13)  RndMeth=Convergent  SaturateOnIntegerOverflow=on  SampleTime=1
  a(3)(1) : Gain  Gain="fi(0,0,16,16,\"hex\",\"ea3c\")"  ParamDataTypeStr=fixdt(0, 16, 16)  OutDataTypeStr=fixdt(1, 32, 14)  RndMeth=Convergent  SaturateOnIntegerOverflow=on  SampleTime=1
  b(2)(1) : Gain  Gain="fi(0,1,16,14,\"hex\",\"8000\")"  ParamDataTypeStr=fixdt(1, 16, 14)  OutDataTypeStr=fixdt(1, 32, 13)  RndMeth=Convergent  SaturateOnIntegerOverflow=on  SampleTime=1
  s(1) : Gain  Gain="fi(0,0,16,16,\"hex\",\"f4e0\")"  ParamDataTypeStr=fixdt(0, 16, 16)  OutDataTypeStr=fixdt(1, 16, 4)  RndMeth=Convergent  SaturateOnIntegerOverflow=on  SampleTime=1
  t : Demux  Outputs=2
  Output : Outport  InitialOutput=0
  Output1 : Outport  Port=2  InitialOutput=0
  wires:
  t/2 -> Input1_1_wire/1
  t/1 -> Input1_0_wire/1
  s(1)/1 -> SumA21/1
  b(2)(1)/1 -> SumB21/2
  a(3)(1)/1 -> SumA31/2
  a(2)(1)/1 -> SumA21/2
  SumB31/1 -> ConvertOut/1
  SumB21/1 -> SumB31/1
  SumA31/1 -> CastState1/1
  SumA21/1 -> SumA31/1
  Input1_1_wire/1 -> a(2)(1)/1, b(2)(1)/1
  Input1_0_wire/1 -> a(3)(1)/1, SumB31/2
  ConvertOut/1 -> Output/1
  ConvertIn/1 -> s(1)/1
  CastState1/1 -> Output1/1, SumB21/1
  Input1/1 -> t/1
  Input/1 -> ConvertIn/1

== system gm_CustArch_v7_vnl/cust_architecture/process_and_retrieve/previous_sample_storage2/PreviousData_read ==
  u2 : Inport  OutDataTypeStr=fixdt(0, 9, 0)  PortDimensions=1  SampleTime=1
  Enable : EnablePort  OutDataTypeStr=boolean
  1st1 : Constant  OutDataTypeStr=boolean  SampleTime=1
  Bit Concat1 : hdlsllib/Logic and Bit Operations/Bit Concat  numInputs=2
  y : Outport  InitialOutput=0
  wires:
  Bit Concat1/1 -> y/1
  1st1/1 -> Bit Concat1/1
  u2/1 -> Bit Concat1/2

== system gm_CustArch_v7_vnl/cust_architecture_vnl/collect_output/read_from_magic_and_timestamp/getting address and enable for Magic and Timestamps ==
  note: enable the RAM writing if the InputState is between 0 and 5
  note: LETìS REPLACE THIS SHIT (WHICH WORKS) WITH A MATLAB FUNCTION
  note: this associates a RAM address to the magic number and timestamp
      | data according to the InputState
      |
      | InputState from 0 to 5 for magic number and timestamp
  InputState : Inport
  FIFO_write_to : Inport  Port=2
  AND1 : Logic  IconShape=distinctive  AllPortsSameDT=off  OutDataTypeStr=boolean
  Compare To Constant10 : simulink/Logic and Bit Operations/Compare To Constant  relop===  const=4  OutDataTypeStr=boolean
  Compare To Constant11 : simulink/Logic and Bit Operations/Compare To Constant  relop===  const=5  OutDataTypeStr=boolean
  Compare To Constant12 : simulink/Logic and Bit Operations/Compare To Constant  relop=<=  const=5  OutDataTypeStr=boolean
  Compare To Constant6 : simulink/Logic and Bit Operations/Compare To Constant  relop===  const=0  OutDataTypeStr=boolean
  Compare To Constant7 : simulink/Logic and Bit Operations/Compare To Constant  relop===  const=1  OutDataTypeStr=boolean
  Compare To Constant8 : simulink/Logic and Bit Operations/Compare To Constant  relop===  const=2  OutDataTypeStr=boolean
  Compare To Constant9 : simulink/Logic and Bit Operations/Compare To Constant  relop===  const=3  OutDataTypeStr=boolean
  Constant10 : Constant  Value=3  OutDataTypeStr=uint8  SampleTime=-1
  Constant11 : Constant  Value=4  OutDataTypeStr=uint8  SampleTime=-1
  Constant12 : Constant  Value=5  OutDataTypeStr=uint8  SampleTime=-1
  Constant13 : Constant  Value=6  OutDataTypeStr=uint8  SampleTime=-1
  Constant7 : Constant  Value=0  OutDataTypeStr=uint8  SampleTime=-1
  Constant8 : Constant  OutDataTypeStr=uint8  SampleTime=-1
  Constant9 : Constant  Value=2  OutDataTypeStr=uint8  SampleTime=-1
  Switch{6..11} (6 alike) : Switch  Criteria=u2 > Threshold
  wr_address : Outport  VectorParamsAs1DForOutWhenUnconnected=off
  wr_enable : Outport  Port=2  VectorParamsAs1DForOutWhenUnconnected=off
  wires:
  Switch9/1 -> Switch8/3
  Compare To Constant10/1 -> Switch10/2
  Switch7/1 -> Switch6/3
  Constant13/1 -> Switch11/3
  Switch8/1 -> Switch7/3
  Constant8/1 -> Switch7/1
  Constant12/1 -> Switch11/1
  Compare To Constant11/1 -> Switch11/2
  Constant7/1 -> Switch6/1
  Switch6/1 -> wr_address/1
  Constant11/1 -> Switch10/1
  Switch11/1 -> Switch10/3
  InputState/1 -> Compare To Constant6/1, Compare To Constant7/1, Compare To Constant8/1, Compare To Constant9/1, Compare To Constant11/1, Compare To Constant12/1, Compare To Constant10/1
  FIFO_write_to/1 -> AND1/2
  Compare To Constant6/1 -> Switch6/2
  Constant9/1 -> Switch8/1
  Compare To Constant12/1 -> AND1/1
  Switch10/1 -> Switch9/3
  Compare To Constant9/1 -> Switch9/2
  AND1/1 -> wr_enable/1
  Compare To Constant7/1 -> Switch7/2
  Compare To Constant8/1 -> Switch8/2
  Constant10/1 -> Switch9/1

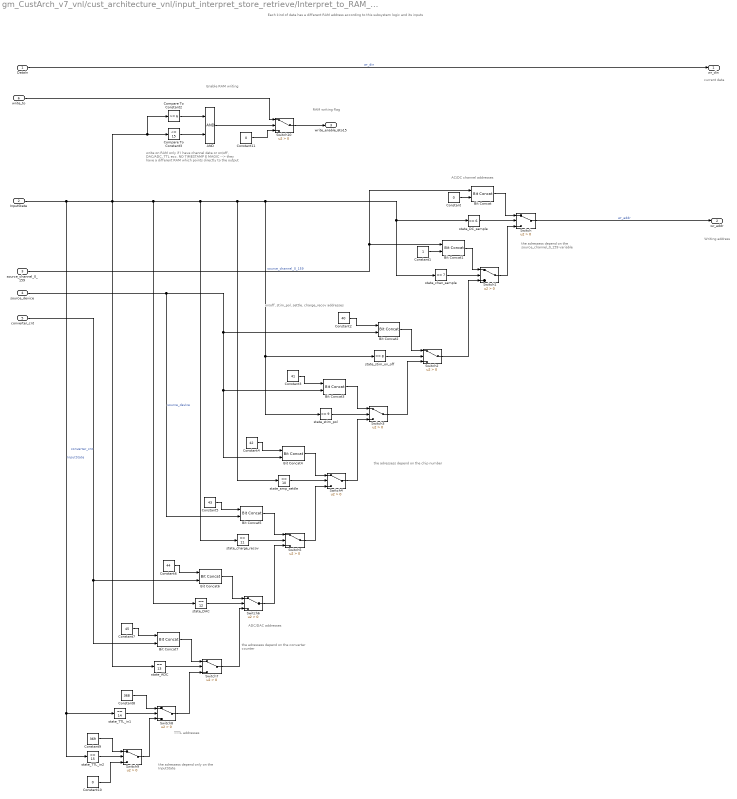
== system gm_CustArch_v7_vnl/cust_architecture_vnl/input_interpret_store_retrieve/Interpret_to_RAM_input/RAM address definition ==
  note: Enable RAM writing
  note: the adressess depend on the
      | source_channel_0_159 variable
  note: the adressess depend only on the
      | InputState
  note: the adressess depend on the converter
      | counter
  note: TTTL addresses
  note: ADC/DAC addresses
  note: on/off, stim_pol, settle, charge_recov addresses
  note: write on RAM only if I have channel data or on/off,
      | DAC/ADC, TTL ecc.
      | NO TIMESTAMP E MAGIC --> they have a different
      | RAM which points directly to the output
  note: RAM writing flag
  note: current data
  note: Writing address
  note: AC/DC channel addresses
  note: Each kind of data has a different RAM
      | address according to this subsystem logic
      | and its inputs
  note: the adressess depend on the chip number
  DataIn : Inport
  InputState : Inport  Port=2
  source_channel_0_159 : Inport  Port=3
  source_device : Inport  Port=4
  converter_cnt : Inport  Port=5
  write_to : Inport  Port=6  OutDataTypeStr=boolean
  AND : Logic  IconShape=distinctive  AllPortsSameDT=off  OutDataTypeStr=boolean
  Bit Concat{,1..7} (8 alike) : hdlsllib/Logic and Bit Operations/Bit Concat  numInputs=2
  Compare To Constant2 : simulink/Logic and Bit Operations/Compare To Constant  relop=>=  const=6  OutDataTypeStr=boolean
  Compare To Constant3 : simulink/Logic and Bit Operations/Compare To Constant  relop=<=  const=15  OutDataTypeStr=boolean
  Constant : Constant  Value=0  OutDataTypeStr=boolean  SampleTime=-1
  Constant1 : Constant  OutDataTypeStr=boolean  SampleTime=-1
  Constant10 : Constant  Value=0  OutDataTypeStr=fixdt(0,9)  SampleTime=-1
  Constant11 : Constant  Value=0  OutDataTypeStr=boolean  SampleTime=-1
  Constant2 : Constant  Value=40  OutDataTypeStr=fixdt(0,6)  SampleTime=-1
  Constant3 : Constant  Value=41  OutDataTypeStr=fixdt(0,6)  SampleTime=-1
  Constant4 : Constant  Value=42  OutDataTypeStr=fixdt(0,6)  SampleTime=-1
  Constant5 : Constant  Value=43  OutDataTypeStr=fixdt(0,6)  SampleTime=-1
  Constant6 : Constant  Value=44  OutDataTypeStr=fixdt(0,6)  SampleTime=-1
  Constant7 : Constant  Value=45  OutDataTypeStr=fixdt(0,6)  SampleTime=-1
  Constant8 : Constant  Value=368  OutDataTypeStr=fixdt(0,9)  SampleTime=-1
  Constant9 : Constant  Value=369  OutDataTypeStr=fixdt(0,9)  SampleTime=-1
  Switch{,1..10} (11 alike) : Switch  Criteria=u2 > Threshold
  state_ADC : simulink/Logic and Bit Operations/Compare To Constant  relop===  const=13  OutDataTypeStr=boolean
  state_DAC : simulink/Logic and Bit Operations/Compare To Constant  relop===  const=12  OutDataTypeStr=boolean
  state_DC_sample : simulink/Logic and Bit Operations/Compare To Constant  relop===  const=6  OutDataTypeStr=boolean
  state_TTL_in1 : simulink/Logic and Bit Operations/Compare To Constant  relop===  const=14  OutDataTypeStr=boolean
  state_TTL_in2 : simulink/Logic and Bit Operations/Compare To Constant  relop===  const=15  OutDataTypeStr=boolean
  state_amp_settle : simulink/Logic and Bit Operations/Compare To Constant  relop===  const=10  OutDataTypeStr=boolean
  state_chan_sample : simulink/Logic and Bit Operations/Compare To Constant  relop===  const=7  OutDataTypeStr=boolean
  state_charge_recov : simulink/Logic and Bit Operations/Compare To Constant  relop===  const=11  OutDataTypeStr=boolean
  state_stim_on_off : simulink/Logic and Bit Operations/Compare To Constant  relop===  const=8  OutDataTypeStr=boolean
  state_stim_pol : simulink/Logic and Bit Operations/Compare To Constant  relop===  const=9  OutDataTypeStr=boolean
  wr_din : Outport  VectorParamsAs1DForOutWhenUnconnected=off
  wr_addr : Outport  Port=2  OutDataTypeStr=fixdt(0,9,0)  VectorParamsAs1DForOutWhenUnconnected=off
  write_enable_6to15 : Outport  Port=3  OutDataTypeStr=boolean  VectorParamsAs1DForOutWhenUnconnected=off
  wires:
  Constant11/1 -> Switch10/3
  Compare To Constant2/1 -> AND/1
  write_to/1 -> Switch10/1
  Switch10/1 -> write_enable_6to15/1
  AND/1 -> Switch10/2
  InputState/1 -> Compare To Constant3/1, Compare To Constant2/1, state_DC_sample/1, state_chan_sample/1, state_stim_on_off/1, state_stim_pol/1, state_amp_settle/1, state_charge_recov/1, state_DAC/1, state_ADC/1, state_TTL_in2/1, state_TTL_in1/1  "InputState"
  Compare To Constant3/1 -> AND/2
  DataIn/1 -> wr_din/1  "wr_din"
  Constant10/1 -> Switch9/3
  Switch9/1 -> Switch8/3
  Constant9/1 -> Switch9/1
  state_TTL_in2/1 -> Switch9/2
  Switch8/1 -> Switch7/3
  Constant8/1 -> Switch8/1
  state_TTL_in1/1 -> Switch8/2
  Switch7/1 -> Switch6/3
  Constant7/1 -> Bit Concat7/1
  state_ADC/1 -> Switch7/2
  Bit Concat7/1 -> Switch7/1
  converter_cnt/1 -> Bit Concat6/2, Bit Concat7/2  "converter_cnt"
  Switch6/1 -> Switch5/3
  Constant6/1 -> Bit Concat6/1
  state_DAC/1 -> Switch6/2
  Bit Concat6/1 -> Switch6/1
  Switch5/1 -> Switch4/3
  source_device/1 -> Bit Concat2/2, Bit Concat3/2, Bit Concat4/2, Bit Concat5/2  "source_device"
  Constant5/1 -> Bit Concat5/1
  state_charge_recov/1 -> Switch5/2
  Bit Concat5/1 -> Switch5/1
  Switch4/1 -> Switch3/3
  Bit Concat4/1 -> Switch4/1
  state_amp_settle/1 -> Switch4/2
  Constant4/1 -> Bit Concat4/1
  Switch3/1 -> Switch2/3
  Bit Concat3/1 -> Switch3/1
  state_stim_pol/1 -> Switch3/2
  Constant3/1 -> Bit Concat3/1
  Switch2/1 -> Switch1/3
  state_stim_on_off/1 -> Switch2/2
  Bit Concat2/1 -> Switch2/1
  Constant2/1 -> Bit Concat2/1
  Switch/1 -> wr_addr/1  "wr_addr"
  Switch1/1 -> Switch/3
  Bit Concat1/1 -> Switch1/1
  Constant1/1 -> Bit Concat1/2
  state_chan_sample/1 -> Switch1/2
  Bit Concat/1 -> Switch/1
  Constant/1 -> Bit Concat/2
  source_channel_0_159/1 -> Bit Concat/1, Bit Concat1/1  "source_channel_0_159"
  state_DC_sample/1 -> Switch/2

== system gm_CustArch_v7_vnl/cust_architecture_vnl/input_interpret_store_retrieve/Interpret_to_RAM_input/interpret incoming data ==
  note: necessary to move
      | forward from state 6 to 8
  note: channel (electrode) under
      | processing
  note: channel data
      | address
  note: amplifier chip under
      | processing
  note: to reduce the number of bit to encode
      | the soure device since it could takes
      | values from 0 to 7
  note: ADC/DAC counter
      | (from 0 to 7 for each)
  note: check ADC/DAC state
  note: to reduce the number of bit to encode
      | the ADC/DAC counter since it could takes
      | values from 0 to 7
  note: counter of the converters
  FIFO_write_to : Inport
  InputState : Inport  Port=2
  data_stream_enable : Inport  Port=3
  Bit Slice : hdlsllib/Logic and Bit Operations/Bit Slice  lidx=2  ridx=0
      settings: SourceProductBaseCode=SL
  Bit Slice1 : hdlsllib/Logic and Bit Operations/Bit Slice  lidx=2  ridx=0
      settings: SourceProductBaseCode=SL
  HDL Counter : hdlsllib/Sources/HDL Counter  CountType=Count limited  CountInit=0  CountStep=1  CountMax=7  CountFromType=Specify  CountFrom=0  CountResetPort=off  CountLoadPort=off  CountEnbPort=on  CountDirPort=off  CountDataType=Unsigned  CountWordLen=8  CountFracLen=0  CountSampTime=1
  "condition to count DAC or ADC " : Subsystem
  get_sources_and_RAM_addresses : Subsystem
  source_device : Outport  VectorParamsAs1DForOutWhenUnconnected=off
  inc_source_device : Outport  Port=2  VectorParamsAs1DForOutWhenUnconnected=off
  device_output : Outport  Port=3  VectorParamsAs1DForOutWhenUnconnected=off
  source_channel_0_159 : Outport  Port=4  VectorParamsAs1DForOutWhenUnconnected=off
  converter_cnt : Outport  Port=5  VectorParamsAs1DForOutWhenUnconnected=off
  wires:
  get_sources_and_RAM_addresses/4(inc_source_device) -> inc_source_device/1
  Bit Slice1/1 -> source_device/1
  get_sources_and_RAM_addresses/2(device_output) -> device_output/1
  get_sources_and_RAM_addresses/3(source_channel) -> source_channel_0_159/1
  get_sources_and_RAM_addresses/1(source_device) -> Bit Slice1/1
  HDL Counter/1 -> Bit Slice/1
  Bit Slice/1 -> converter_cnt/1
  "condition to count DAC or ADC "/1(Out1) -> HDL Counter/1
  InputState/1 -> get_sources_and_RAM_addresses/2(InputState), "condition to count DAC or ADC "/2(input_state)
  data_stream_enable/1 -> get_sources_and_RAM_addresses/3(data_stream_enable)
  FIFO_write_to/1 -> get_sources_and_RAM_addresses/1(FIFO_write_to), "condition to count DAC or ADC "/1(fifo_write_to)
